simulink model "third_28_02_25"  (R2022b)
settings: Solver=VariableStepAuto  StartTime=0.0  StopTime=10.0  MaxStep=1e-5  RelTol=1e-3
undefined symbols (not defined in the file): fsw, l, r
libraries: simulink x2
settings Model: Creator=claudio.rossi  LastModifiedBy=claudio.rossi

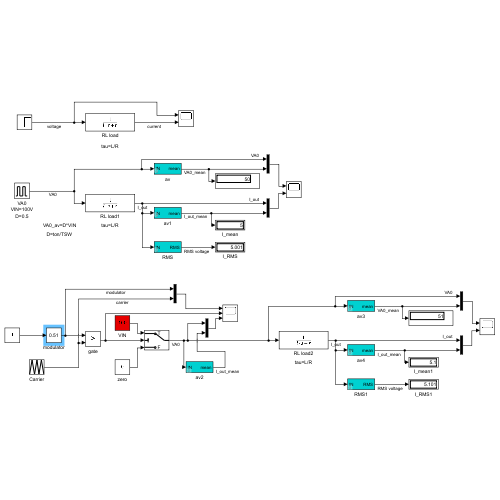
[thumbnail: Simulink's stored preview of the top-level diagram]
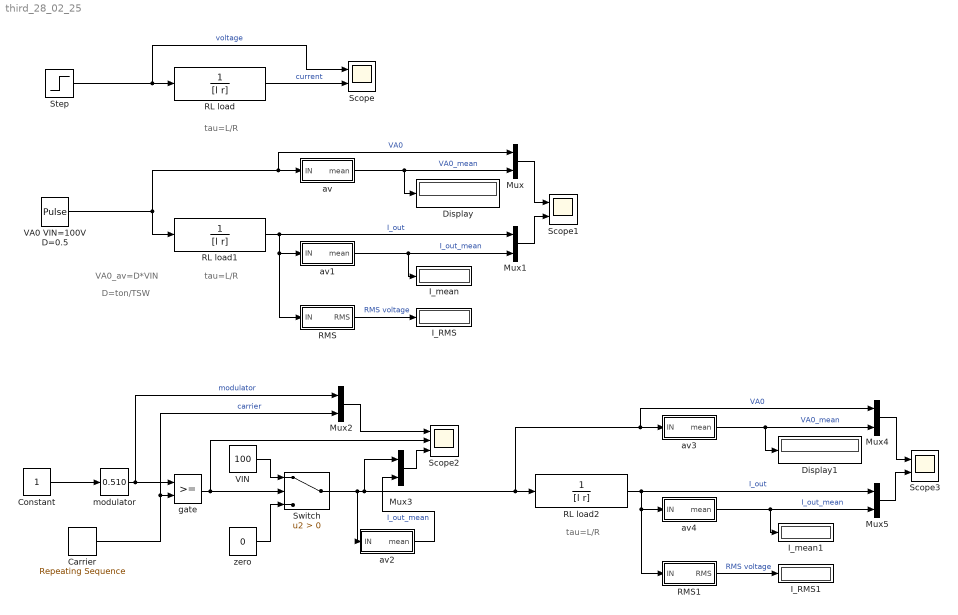
== system third_28_02_25 ==
  note: VA0_av=D*VIN
  note: D=ton/TSW
  note: tau=L/R
  note: tau=L/R
  note: tau=L/R
  "Carrier " : simulink/Sources/Repeating Sequence  rep_seq_t=[0 0.5/fsw 1/fsw]  rep_seq_y=[0 1 0 ]
  Constant : Constant
  Display : Display
  Display1 : Display
  I_RMS : Display
  I_RMS1 : Display
  I_mean : Display
  I_mean1 : Display
  Mux{,1..5} (6 alike) : Mux  Inputs=2
  RL load : TransferFcn  Denominator=[l r]
  RL load1 : TransferFcn  Denominator=[l r]
  RL load2 : TransferFcn  Denominator=[l r]
  RMS : Subsystem  mask{period=1/fsw}
      mask prompts: period "period [s]"
      mask DialogControl DescTextVar Prompt: calculates the RMS of a periodic function with period specified here
  RMS1 : Subsystem  mask{period=1/fsw}
      mask prompts: period "period [s]"
      mask DialogControl DescTextVar Prompt: calculates the RMS of a periodic function with period specified here
  Scope : Scope  NumInputPorts=2
  Scope1 : Scope  NumInputPorts=2
  Scope2 : Scope  NumInputPorts=3
  Scope3 : Scope  NumInputPorts=2
  Step : Step  After=100  SampleTime=0
  Switch : Switch  Criteria=u2 > Threshold  SaturateOnIntegerOverflow=off  InputSameDT=off
  VA0 VIN=100V D=0.5 : DiscretePulseGenerator  PulseType=Time based  Amplitude=100  Period=1/fsw  PulseWidth=50
  VIN : Constant  Value=100
  av : Subsystem  mask{period=1/fsw}
      mask prompts: period "period [s]"
      mask DialogControl DescTextVar Prompt: calculate the averge over period
      mask DialogControl text Prompt: test
  av1 : Subsystem  mask{period=1/fsw}
      mask prompts: period "period [s]"
      mask DialogControl DescTextVar Prompt: calculate the averge over period
      mask DialogControl text Prompt: test
  av2 : Subsystem  mask{period=1/fsw}
      mask prompts: period "period [s]"
      mask DialogControl DescTextVar Prompt: calculate the averge over period
      mask DialogControl text Prompt: test
  av3 : Subsystem  mask{period=1/fsw}
      mask prompts: period "period [s]"
      mask DialogControl DescTextVar Prompt: calculate the averge over period
      mask DialogControl text Prompt: test
  av4 : Subsystem  mask{period=1/fsw}
      mask prompts: period "period [s]"
      mask DialogControl DescTextVar Prompt: calculate the averge over period
      mask DialogControl text Prompt: test
  gate : RelationalOperator  OutDataTypeStr=boolean  RndMeth=Simplest  InputSameDT=off
  modulator : simulink/Math Operations/Slider Gain  gain=0.510  low=0  high=1
  zero : Constant  Value=0
  wires:
  Step/1 -> Scope/1, RL load/1  "voltage"
  RL load/1 -> Scope/2  "current"
  VA0 VIN=100V D=0.5/1 -> RL load1/1, Mux/1, av/1(IN)  "VA0"
  av/1(mean) -> Display/1, Mux/2  "VA0_mean"
  Mux/1 -> Scope1/1
  av1/1(mean) -> I_mean/1, Mux1/2  "I_out_mean"
  Mux1/1 -> Scope1/2
  RL load1/1 -> Mux1/1, RMS/1(IN), av1/1(IN)  "I_out"
  RMS/1(RMS) -> I_RMS/1  "RMS voltage"
  "Carrier "/1 -> Mux2/2, gate/2  "carrier"
  Constant/1 -> modulator/1
  modulator/1 -> Mux2/1, gate/1  "modulator"
  gate/1 -> Switch/2, Scope2/2
  VIN/1 -> Switch/1
  zero/1 -> Switch/3
  Mux2/1 -> Scope2/1
  Mux3/1 -> Scope2/3
  Switch/1 -> av2/1(IN), av3/1(IN), Mux4/1, RL load2/1, Mux3/1  "VA0"
  av2/1(mean) -> Mux3/2  "I_out_mean"
  RMS1/1(RMS) -> I_RMS1/1  "RMS voltage"
  RL load2/1 -> av4/1(IN), RMS1/1(IN), Mux5/1  "I_out"
  Mux5/1 -> Scope3/2
  av4/1(mean) -> Mux5/2, I_mean1/1  "I_out_mean"
  Mux4/1 -> Scope3/1
  av3/1(mean) -> Mux4/2, Display1/1  "VA0_mean"

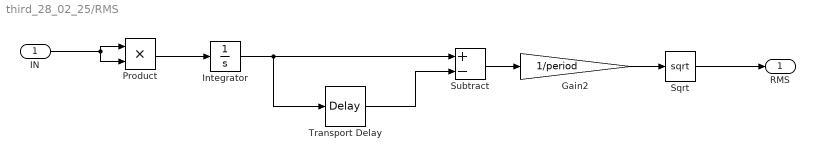
== system third_28_02_25/RMS ==
  IN : Inport
  Gain2 : Gain  Gain=1/period
  Integrator : Integrator
  Product : Product
  Sqrt : Sqrt
  Subtract : Sum  Inputs=+-
  Transport Delay : TransportDelay  DelayTime=period
  RMS : Outport
  wires:
  Sqrt/1 -> RMS/1
  Gain2/1 -> Sqrt/1
  Product/1 -> Integrator/1
  IN/1 -> Product/2, Product/1
  Integrator/1 -> Transport Delay/1, Subtract/1
  Subtract/1 -> Gain2/1
  Transport Delay/1 -> Subtract/2

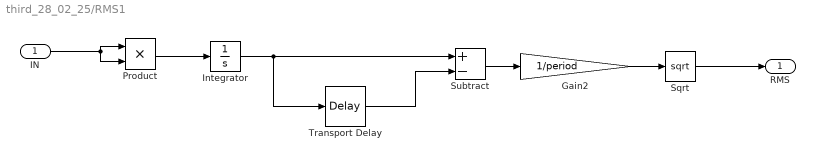
== system third_28_02_25/RMS1 ==
  IN : Inport
  Gain2 : Gain  Gain=1/period
  Integrator : Integrator
  Product : Product
  Sqrt : Sqrt
  Subtract : Sum  Inputs=+-
  Transport Delay : TransportDelay  DelayTime=period
  RMS : Outport
  wires:
  Transport Delay/1 -> Subtract/2
  Subtract/1 -> Gain2/1
  Integrator/1 -> Subtract/1, Transport Delay/1
  IN/1 -> Product/1, Product/2
  Product/1 -> Integrator/1
  Gain2/1 -> Sqrt/1
  Sqrt/1 -> RMS/1

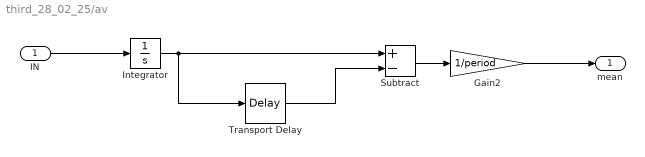
== system third_28_02_25/av ==
  IN : Inport
  Gain2 : Gain  Gain=1/period
  Integrator : Integrator
  Subtract : Sum  Inputs=+-
  Transport Delay : TransportDelay  DelayTime=period
  mean : Outport
  wires:
  Integrator/1 -> Transport Delay/1, Subtract/1
  Gain2/1 -> mean/1
  Subtract/1 -> Gain2/1
  Transport Delay/1 -> Subtract/2
  IN/1 -> Integrator/1

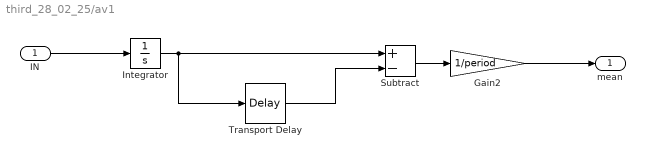
== system third_28_02_25/av1 ==
  IN : Inport
  Gain2 : Gain  Gain=1/period
  Integrator : Integrator
  Subtract : Sum  Inputs=+-
  Transport Delay : TransportDelay  DelayTime=period
  mean : Outport
  wires:
  IN/1 -> Integrator/1
  Transport Delay/1 -> Subtract/2
  Subtract/1 -> Gain2/1
  Gain2/1 -> mean/1
  Integrator/1 -> Subtract/1, Transport Delay/1

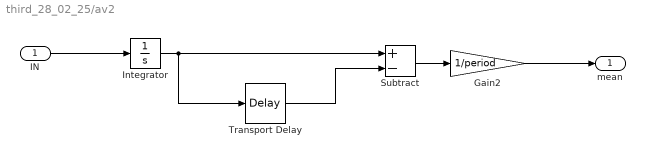
== system third_28_02_25/av2 ==
  IN : Inport
  Gain2 : Gain  Gain=1/period
  Integrator : Integrator
  Subtract : Sum  Inputs=+-
  Transport Delay : TransportDelay  DelayTime=period
  mean : Outport
  wires:
  Integrator/1 -> Transport Delay/1, Subtract/1
  Gain2/1 -> mean/1
  Subtract/1 -> Gain2/1
  Transport Delay/1 -> Subtract/2
  IN/1 -> Integrator/1

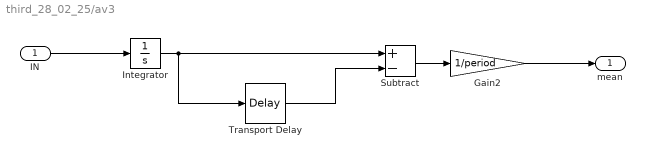
== system third_28_02_25/av3 ==
  IN : Inport
  Gain2 : Gain  Gain=1/period
  Integrator : Integrator
  Subtract : Sum  Inputs=+-
  Transport Delay : TransportDelay  DelayTime=period
  mean : Outport
  wires:
  IN/1 -> Integrator/1
  Transport Delay/1 -> Subtract/2
  Subtract/1 -> Gain2/1
  Gain2/1 -> mean/1
  Integrator/1 -> Subtract/1, Transport Delay/1

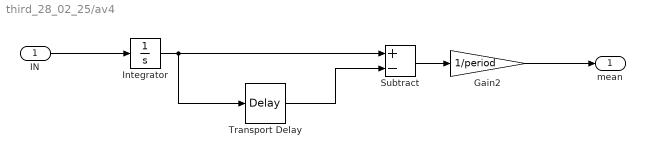
== system third_28_02_25/av4 ==
  IN : Inport
  Gain2 : Gain  Gain=1/period
  Integrator : Integrator
  Subtract : Sum  Inputs=+-
  Transport Delay : TransportDelay  DelayTime=period
  mean : Outport
  wires:
  Integrator/1 -> Transport Delay/1, Subtract/1
  Gain2/1 -> mean/1
  Subtract/1 -> Gain2/1
  Transport Delay/1 -> Subtract/2
  IN/1 -> Integrator/1
